simulink model "EISGov_TrqLosEst"  (R2016b)
settings: configuration reference "CodeGenConfigSet" (kept outside this file)
values from neighbouring files (symbols this model uses):
  EISGov_dnEngFltIni_C = Calibration.Parameter    [init_EISGov_TrqLosEst.m]    (also in init_EISGov_TrqLosEst_SIL.m = Simulink.Parameter)
  EISGov_facdnAccDecLim_CUR = Calibration.Parameter    [init_EISGov_TrqLosEst.m]    (also in init_EISGov_TrqLosEst_SIL.m = Simulink.Parameter)
  EISGov_facdnAccDecLim_CURX = Calibration.Parameter    [init_EISGov_TrqLosEst.m]    (also in init_EISGov_TrqLosEst_SIL.m = Simulink.Parameter)
  EISGov_facEngDnFlt_CUR = Calibration.Parameter    [init_EISGov_TrqLosEst.m]    (also in init_EISGov_TrqLosEst_SIL.m = Simulink.Parameter)
  EISGov_facEngDnFlt_CURX = Calibration.Parameter    [init_EISGov_TrqLosEst.m]    (also in init_EISGov_TrqLosEst_SIL.m = Simulink.Parameter)
  EISGov_swtTempSel_C = Calibration.Parameter    [init_EISGov_TrqLosEst.m]    (also in init_EISGov_TrqLosEst_SIL.m = Simulink.Parameter)
  EISGov_tiSetTimeAccDecLim_CUR = Calibration.Parameter    [init_EISGov_TrqLosEst.m]    (also in init_EISGov_TrqLosEst_SIL.m = Simulink.Parameter)
  EISGov_tiSetTimeAccDecLim_CURX = Calibration.Parameter    [init_EISGov_TrqLosEst.m]    (also in init_EISGov_TrqLosEst_SIL.m = Simulink.Parameter)
  EISGov_titrqLosFlt_C = Calibration.Parameter    [init_EISGov_TrqLosEst.m]    (also in init_EISGov_TrqLosEst_SIL.m = Simulink.Parameter)
  EISGov_trqLosEstSlect_C = Calibration.Parameter    [init_EISGov_TrqLosEst.m]    (also in init_EISGov_TrqLosEst_SIL.m = Simulink.Parameter)
  EISGov_trqLossLimMax_C = Calibration.Parameter    [init_EISGov_TrqLosEst.m]    (also in init_EISGov_TrqLosEst_SIL.m = Simulink.Parameter)
undefined symbols (not defined in the file or in its folder): EngState_conv, HLSDem_KpCorFac_MAPX
libraries: CXLib x5
settings Model: Creator=Administrator  LastModifiedBy=xuxingpei
settings ConfigSetRef: SourceLocation=Base Workspace

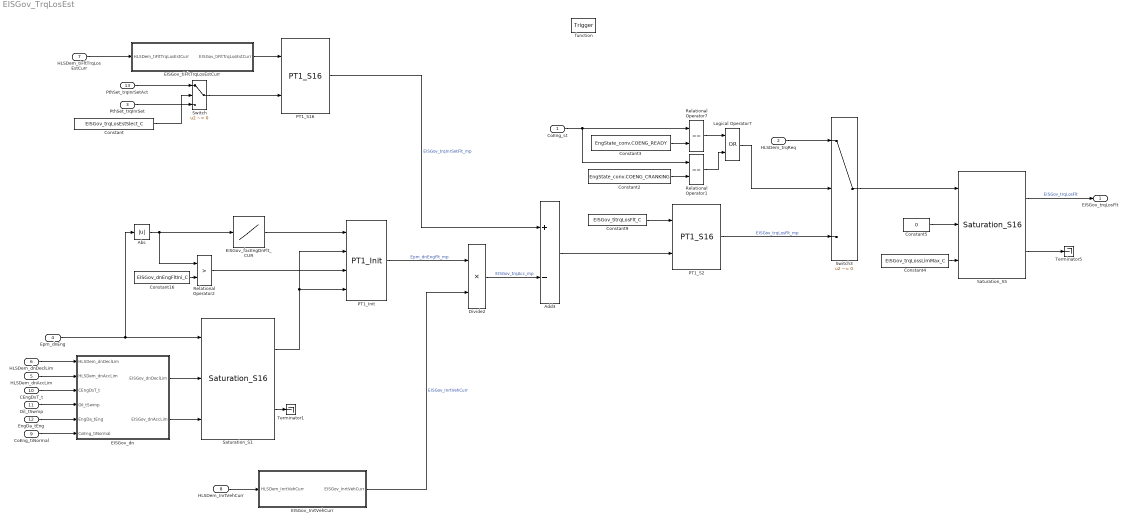
== system EISGov_TrqLosEst ==
  CoEng_st : Inport  Description=Engine coordinator state  OutDataTypeStr=Enum: EngState_conv
  HLSDem_trqReq : Inport  Tag=Nm  Description=Requested initialisation torque to engine speed governor (with reference to the output)  Port=2  OutMin=-3000  OutMax=3000  OutDataTypeStr=Trq_Nm
  PthSet_trqInrSet : Inport  Tag=Nm  Description=Inner torque set value after monitoring limitation  Port=3  OutMin=-3000  OutMax=3276.7  OutDataTypeStr=Trq_Nm
  Epm_dnEng : Inport  Tag=rpm/s  Description=Engine speed gradient calculated over current crankshaft-segment (S0-S0 or S1-S1)  Port=4  OutMin=-12000  OutMax=12000  OutDataTypeStr=EngSpeed_rpm_s
  HLSDem_dnAccLim : Inport  Tag=rpm/s  Description=Maximum permissible acceleration (Engine speed)  Port=5  OutMin=-12000  OutMax=12000  OutDataTypeStr=EngSpeed_rpm_s
  HLSDem_dnDeclLim : Inport  Tag=rpm/s  Description=Maximum permissible deceleration (Engine speed)  Port=6  OutMin=-12000  OutMax=12000  OutDataTypeStr=EngSpeed_rpm_s
  HLSDem_tiFltTrqLosEstCurr : Inport  Description=Time constant (PT1filter) for EISGov torque loss estimation  Port=7  OutMin=0  OutMax=99.998  OutDataTypeStr=PT_fac
  HLSDem_InrtVehCurr : Inport  Tag=Nm/(rpm/s)  Description=Mass Inertia for EISGov torque loss estimation  Port=8  OutMin=-50  OutMax=50  OutDataTypeStr=HLSDem_Inrt
  CoEng_tiNormal : Inport  Tag=ms  Description="Time since state\"CONENG_RUNNING\"was reached"  Port=9  OutMin=0  OutMax=42949672950  OutDataTypeStr=EngTime_ms
  CEngDsT_t : Inport  Tag=deg  Description=engine coolant temperature after filter  Port=10  OutMin=-200  OutMax=200  OutDataTypeStr=Temp_deg
  Oil_tSwmp : Inport  Tag=deg  Description=Oil temperature in oil sump  Port=11  OutMin=-50  OutMax=200  OutDataTypeStr=Temp_deg
  EngDa_tEng : Inport  Tag=deg  Description=Engine temperature  Port=12  OutMin=-1000  OutMax=1000  OutDataTypeStr=Temp_deg
  PthSet_trqInrSetAct : Inport  Tag=Nm  Description=Current inner engine torque  Port=13  OutMin=-3276.8  OutMax=3276.7  OutDataTypeStr=Trq_Nm
  function : TriggerPort  TriggerType=function-call  VariantControl=Variant
  Abs : Abs
  Add3 : Sum  Inputs=+-  SaturateOnIntegerOverflow=on  InputSameDT=on
  Constant : Constant  Value=EISGov_trqLosEstSlect_C
  Constant16 : Constant  Value=EISGov_dnEngFltIni_C
  Constant2 : Constant  Value=EngState_conv.COENG_CRANKING  OutDataTypeStr=Inherit: Inherit via back propagation
  Constant3 : Constant  Value=EngState_conv.COENG_READY  OutDataTypeStr=Inherit: Inherit via back propagation
  Constant4 : Constant  Value=EISGov_trqLossLimMax_C
  Constant5 : Constant  Value=0  OutDataTypeStr=Inherit: Inherit via back propagation
  Constant9 : Constant  Value=EISGov_titrqLosFlt_C
  Divide2 : Product  Inputs=**  OutDataTypeStr=Inherit: Inherit via back propagation  RndMeth=Round  SaturateOnIntegerOverflow=on
  EISGov_InrtVehCurr : Subsystem
  EISGov_dn : Subsystem
  EISGov_facEngDnFlt_CUR : Lookup_n-D  NumberOfTableDimensions=1  BreakpointsForDimension1=EISGov_facEngDnFlt_CURX  Table=EISGov_facEngDnFlt_CUR  ExtrapMethod=Clip  InternalRulePriority=Speed  OutDataTypeStr=Inherit: Inherit via back propagation  RndMeth=Simplest  SaturateOnIntegerOverflow=on
  EISGov_tiFltTrqLosEstCurr : Subsystem
  Logical Operator7 : Logic  Operator=OR  OutDataTypeStr=boolean
  PT1_Init : CXLib/PT1_Init
  PT1_S16 : CXLib/PT1_S16
  PT1_S2 : CXLib/PT1_S16
  Relational Operator1 : RelationalOperator  Operator===  OutDataTypeStr=boolean  RndMeth=Nearest  InputSameDT=on
  Relational Operator2 : RelationalOperator  Operator=>  OutDataTypeStr=boolean  RndMeth=Simplest  InputSameDT=on
  Relational Operator7 : RelationalOperator  Operator===  OutDataTypeStr=boolean  RndMeth=Nearest  InputSameDT=on
  Saturation_S1 : CXLib/Saturation_S16
  Saturation_S5 : CXLib/Saturation_S16
  Switch : Switch  Criteria=u2 ~= 0
  Switch3 : Switch  Criteria=u2 ~= 0  InputSameDT=on
  Terminator1 : Terminator
  Terminator5 : Terminator
  EISGov_trqLosFlt : Outport  Tag=Nm  Description=estimated torque loss  OutMin=-3276.8  OutMax=3276.7  OutDataTypeStr=Trq_Nm
  wires:
  Constant4/1 -> Saturation_S5/3
  EISGov_tiFltTrqLosEstCurr/1(EISGov_tiFltTrqLosEstCurr) -> PT1_S16/1
  Saturation_S5/1 -> EISGov_trqLosFlt/1  "EISGov_trqLosFlt"
  Saturation_S5/2 -> Terminator5/1
  PT1_S2/1 -> Switch3/3  "EISGov_trqLosFlt_mp"
  Epm_dnEng/1 -> Saturation_S1/1, Abs/1
  Saturation_S1/2 -> Terminator1/1
  PT1_S16/1 -> Add3/1  "EISGov_trqInrSetFlt_mp"
  EISGov_InrtVehCurr/1(EISGov_InrtVehCurr) -> Divide2/2  "EISGov_InrtVehCurr"
  Divide2/1 -> Add3/2  "EISGov_trqAcc_mp"
  Add3/1 -> PT1_S2/2
  HLSDem_trqReq/1 -> Switch3/1
  Constant2/1 -> Relational Operator1/2
  Relational Operator1/1 -> Logical Operator7/2
  Relational Operator7/1 -> Logical Operator7/1
  Constant3/1 -> Relational Operator7/2
  CoEng_st/1 -> Relational Operator1/1, Relational Operator7/1
  Logical Operator7/1 -> Switch3/2
  Switch3/1 -> Saturation_S5/1
  Constant5/1 -> Saturation_S5/2
  EISGov_dn/1(EISGov_dnDeclLim) -> Saturation_S1/2
  EISGov_dn/2(EISGov_dnAccLim) -> Saturation_S1/3
  HLSDem_dnDeclLim/1 -> EISGov_dn/1(HLSDem_dnDeclLim)
  HLSDem_dnAccLim/1 -> EISGov_dn/2(HLSDem_dnAccLim)
  HLSDem_InrtVehCurr/1 -> EISGov_InrtVehCurr/1(HLSDem_InrtVehCurr)
  HLSDem_tiFltTrqLosEstCurr/1 -> EISGov_tiFltTrqLosEstCurr/1(HLSDem_tiFltTrqLosEstCurr)
  CoEng_tiNormal/1 -> EISGov_dn/6(CoEng_tiNormal)
  CEngDsT_t/1 -> EISGov_dn/3(CEngDsT_t)
  Oil_tSwmp/1 -> EISGov_dn/4(Oil_tSwmp)
  EngDa_tEng/1 -> EISGov_dn/5(EngDa_tEng)
  PthSet_trqInrSetAct/1 -> Switch/1
  Switch/1 -> PT1_S16/2
  PthSet_trqInrSet/1 -> Switch/3
  Constant/1 -> Switch/2
  Saturation_S1/1 -> PT1_Init/4, PT1_Init/2
  PT1_Init/1 -> Divide2/1  "Epm_dnEngFlt_mp"
  Constant9/1 -> PT1_S2/1
  Abs/1 -> EISGov_facEngDnFlt_CUR/1, Relational Operator2/1
  Constant16/1 -> Relational Operator2/2
  Relational Operator2/1 -> PT1_Init/3
  EISGov_facEngDnFlt_CUR/1 -> PT1_Init/1

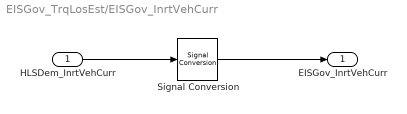
== system EISGov_TrqLosEst/EISGov_InrtVehCurr ==
  HLSDem_InrtVehCurr : Inport
  Signal Conversion : SignalConversion  OverrideOpt=off
  EISGov_InrtVehCurr : Outport
  wires:
  HLSDem_InrtVehCurr/1 -> Signal Conversion/1
  Signal Conversion/1 -> EISGov_InrtVehCurr/1

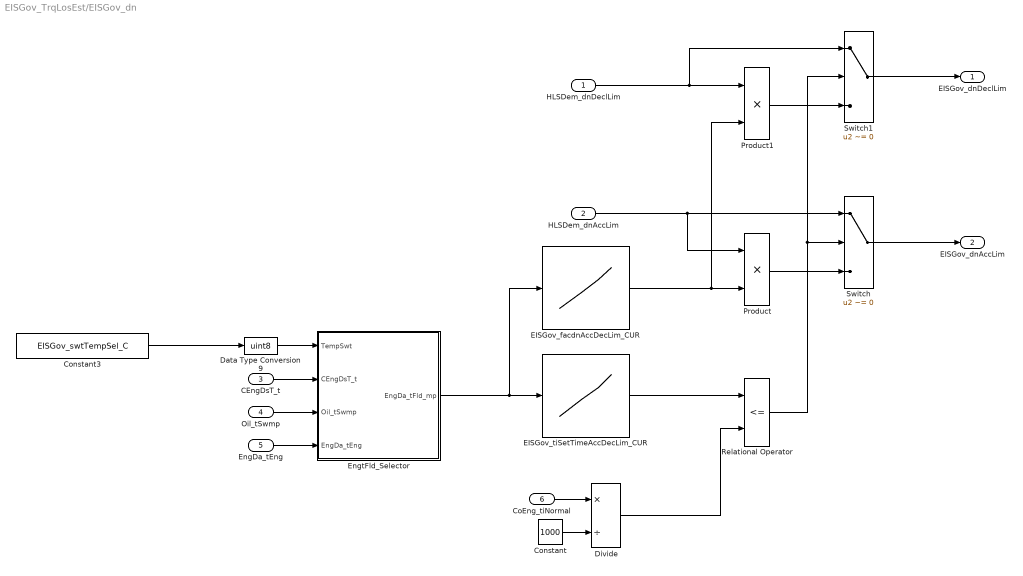
== system EISGov_TrqLosEst/EISGov_dn ==
  HLSDem_dnDeclLim : Inport
  HLSDem_dnAccLim : Inport  Port=2
  CEngDsT_t : Inport  Tag=deg  Description=engine coolant temperature after filter  Port=3  OutMin=-200  OutMax=200  OutDataTypeStr=Temp_deg
  Oil_tSwmp : Inport  Tag=deg  Description=Oil temperature in oil sump  Port=4  OutMin=-50  OutMax=200  OutDataTypeStr=Temp_deg
  EngDa_tEng : Inport  Tag=deg  Description=Engine temperature  Port=5  OutMin=-1000  OutMax=1000  OutDataTypeStr=Temp_deg
  CoEng_tiNormal : Inport  Tag=ms  Description="Time since state\"CONENG_RUNNING\"was reached"  Port=6  OutMin=0  OutMax=42949672950  OutDataTypeStr=EngTime_ms
  Constant : Constant  Value=1000  OutDataTypeStr=Inherit: Inherit via back propagation
  Constant3 : Constant  Value=EISGov_swtTempSel_C
  Data Type Conversion9 : DataTypeConversion  OutDataTypeStr=uint8
  Divide : Product  Inputs=*/  OutDataTypeStr=Inherit: Inherit via back propagation
  EISGov_facdnAccDecLim_CUR : Lookup_n-D  NumberOfTableDimensions=1  BreakpointsForDimension1=EISGov_facdnAccDecLim_CURX  BreakpointsForDimension2=HLSDem_KpCorFac_MAPX  Table=EISGov_facdnAccDecLim_CUR  ExtrapMethod=Clip  InternalRulePriority=Speed  OutDataTypeStr=Inherit: Inherit via back propagation  RndMeth=Simplest  SaturateOnIntegerOverflow=on
  EISGov_tiSetTimeAccDecLim_CUR : Lookup_n-D  NumberOfTableDimensions=1  BreakpointsForDimension1=EISGov_tiSetTimeAccDecLim_CURX  BreakpointsForDimension2=HLSDem_KpCorFac_MAPX  Table=EISGov_tiSetTimeAccDecLim_CUR  ExtrapMethod=Clip  InternalRulePriority=Speed  OutDataTypeStr=Inherit: Inherit via back propagation  RndMeth=Simplest  SaturateOnIntegerOverflow=on
  EngtFld_Selector : Subsystem
  Product : Product  OutDataTypeStr=Inherit: Inherit via back propagation  SaturateOnIntegerOverflow=on
  Product1 : Product  OutDataTypeStr=Inherit: Inherit via back propagation  SaturateOnIntegerOverflow=on
  Relational Operator : RelationalOperator  Operator=<=  OutDataTypeStr=boolean  RndMeth=Simplest  InputSameDT=on
  Switch : Switch  Criteria=u2 ~= 0  InputSameDT=on
  Switch1 : Switch  Criteria=u2 ~= 0  InputSameDT=on
  EISGov_dnDeclLim : Outport
  EISGov_dnAccLim : Outport  Port=2
  wires:
  HLSDem_dnAccLim/1 -> Switch/1, Product/1
  HLSDem_dnDeclLim/1 -> Switch1/1, Product1/1
  Constant3/1 -> Data Type Conversion9/1
  Data Type Conversion9/1 -> EngtFld_Selector/1(TempSwt)
  CEngDsT_t/1 -> EngtFld_Selector/2(CEngDsT_t)
  Oil_tSwmp/1 -> EngtFld_Selector/3(Oil_tSwmp)
  EngDa_tEng/1 -> EngtFld_Selector/4(EngDa_tEng)
  EngtFld_Selector/1(EngDa_tFld_mp) -> EISGov_facdnAccDecLim_CUR/1, EISGov_tiSetTimeAccDecLim_CUR/1
  CoEng_tiNormal/1 -> Divide/1
  Constant/1 -> Divide/2
  EISGov_tiSetTimeAccDecLim_CUR/1 -> Relational Operator/1
  Divide/1 -> Relational Operator/2
  EISGov_facdnAccDecLim_CUR/1 -> Product1/2, Product/2
  Product/1 -> Switch/3
  Switch/1 -> EISGov_dnAccLim/1
  Relational Operator/1 -> Switch1/2, Switch/2
  Product1/1 -> Switch1/3
  Switch1/1 -> EISGov_dnDeclLim/1

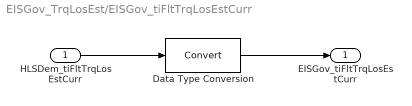
== system EISGov_TrqLosEst/EISGov_tiFltTrqLosEstCurr ==
  HLSDem_tiFltTrqLosEstCurr : Inport
  Data Type Conversion : DataTypeConversion
  EISGov_tiFltTrqLosEstCurr : Outport
  wires:
  HLSDem_tiFltTrqLosEstCurr/1 -> Data Type Conversion/1
  Data Type Conversion/1 -> EISGov_tiFltTrqLosEstCurr/1

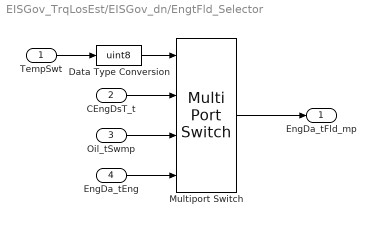
== system EISGov_TrqLosEst/EISGov_dn/EngtFld_Selector ==
  TempSwt : Inport
  CEngDsT_t : Inport  Tag=deg  Description=engine coolant temperature after filter  Port=2
  Oil_tSwmp : Inport  Tag=deg  Description=Oil temperature in oil sump  Port=3
  EngDa_tEng : Inport  Tag=deg  Description=Engine temperature  Port=4
  Data Type Conversion : DataTypeConversion  OutDataTypeStr=uint8
  Multiport Switch : MultiPortSwitch  DataPortOrder=Zero-based contiguous
  EngDa_tFld_mp : Outport  Tag=deg  Description=Engine temperature field
  wires:
  CEngDsT_t/1 -> Multiport Switch/2
  Multiport Switch/1 -> EngDa_tFld_mp/1
  EngDa_tEng/1 -> Multiport Switch/4
  Oil_tSwmp/1 -> Multiport Switch/3
  Data Type Conversion/1 -> Multiport Switch/1
  TempSwt/1 -> Data Type Conversion/1
